simulink model "Aufgabe2"  (R2020a)
settings: Solver=ode4  StartTime=0.0  StopTime=5  FixedStep=1e-3  RelTol=1e-9
undefined symbols (not defined in the file or in its folder): A, A0, A1, B, B0, B1, C, D, J, psi, r, R, x0
settings Model: Creator=Ravi Plenzdorf  LastModifiedBy=Ravi Plenzdorf
settings DataIOCC: ReturnWorkspaceOutputs=off

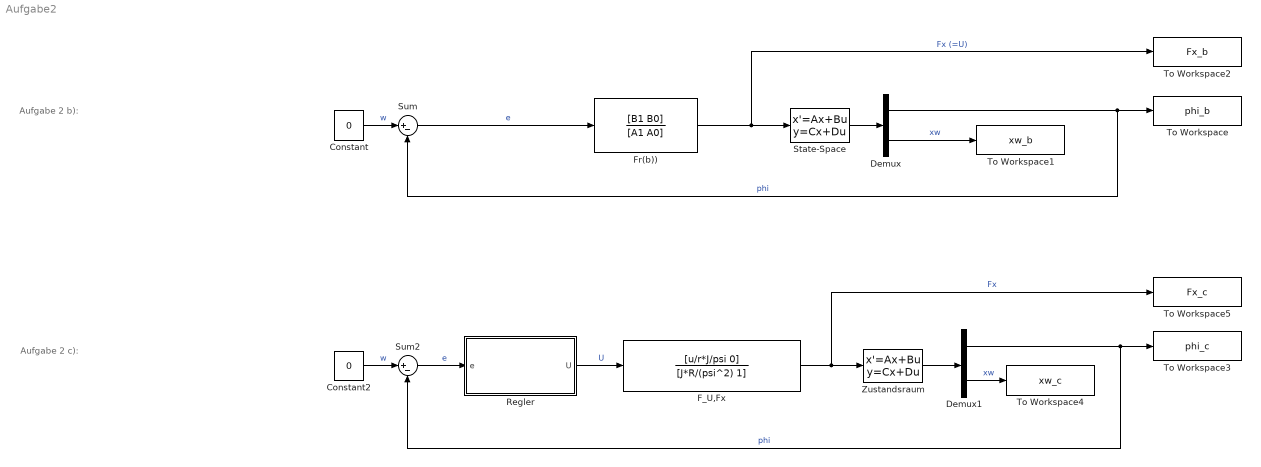
== system Aufgabe2 ==
  note: Aufgabe 2 b):
  note: Aufgabe 2 c):
  Constant : Constant  Value=0
  Constant2 : Constant  Value=0
  Demux : Demux  Outputs=2
  Demux1 : Demux  Outputs=2
  F_U,Fx : TransferFcn  Numerator=[u/r*J/psi 0]  Denominator=[J*R/(psi^2) 1]
  Fr(b)) : TransferFcn  Numerator=[B1 B0]  Denominator=[A1 A0]
  Regler : Subsystem
  State-Space : StateSpace  A=A  B=B  C=C  D=D  InitialCondition=x0
  Sum : Sum  Inputs=|+-
  Sum2 : Sum  Inputs=|+-
  To Workspace : ToWorkspace  VariableName=phi_b  SaveFormat=Timeseries  SampleTime=-1
  To Workspace1 : ToWorkspace  VariableName=xw_b  SaveFormat=Timeseries  SampleTime=-1
  To Workspace2 : ToWorkspace  VariableName=Fx_b  SaveFormat=Timeseries  SampleTime=-1
  To Workspace3 : ToWorkspace  VariableName=phi_c  SaveFormat=Timeseries  SampleTime=-1
  To Workspace4 : ToWorkspace  VariableName=xw_c  SaveFormat=Timeseries  SampleTime=-1
  To Workspace5 : ToWorkspace  VariableName=Fx_c  SaveFormat=Timeseries  SampleTime=-1
  Zustandsraum : StateSpace  A=A  B=B  C=C  D=D  InitialCondition=x0
  wires:
  Constant/1 -> Sum/1  "w"
  Sum/1 -> Fr(b))/1  "e"
  Constant2/1 -> Sum2/1  "w"
  F_U,Fx/1 -> Zustandsraum/1, To Workspace5/1  "Fx"
  Fr(b))/1 -> State-Space/1, To Workspace2/1  "Fx (=U)"
  State-Space/1 -> Demux/1
  Demux/1 -> To Workspace/1, Sum/2  "phi"
  Demux/2 -> To Workspace1/1  "xw"
  Demux1/2 -> To Workspace4/1  "xw"
  Demux1/1 -> Sum2/2, To Workspace3/1  "phi"
  Zustandsraum/1 -> Demux1/1
  Sum2/1 -> Regler/1(e)  "e"
  Regler/1(U) -> F_U,Fx/1  "U"

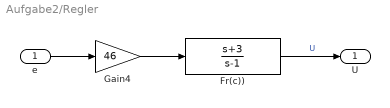
== system Aufgabe2/Regler ==
  e : Inport
  Fr(c)) : TransferFcn  Numerator=[1 +3]  Denominator=[1 -1]
  Gain4 : Gain  Gain=46
  U : Outport
  wires:
  Fr(c))/1 -> U/1  "U"
  Gain4/1 -> Fr(c))/1
  e/1 -> Gain4/1
